simulink model "q_maglev_pid_nominal"  (R2021a)
settings: Solver=ode4  StartTime=0.0  StopTime=inf  FixedStep=5e-4  RelTol=1e-3  AbsTol=1e-6  EnableMultiTasking=on
values from neighbouring files (symbols this model uses):
  IC_MAX = 3    [config_maglev.m]
  K_B = Tb / 4.75    (= 0.00294736842105)    [config_maglev.m]
  Kff_b = ic0 / xb0    [d_maglev_pi_piv.m]
  Ki_c = wn_c^2 * tau_c / Kc_dc    [d_maglev_pi_piv.m]
  Kp_c = (2*zeta_c*wn_c*tau_c - 1) / Kc_dc    [d_maglev_pi_piv.m]
  MAX_XB_WDUP = 1    [setup_maglev.m]
  Rs = 1    [config_maglev.m]
  Tb = 0.014    [config_maglev.m]
  VMAX_AMP = 24    [config_maglev.m]
  xb0 = 6e-3    (= 0.006)    [setup_maglev.m]
  XB_REF_RATE = 5e-3    (= 0.005)    [setup_maglev.m]
undefined symbols (not defined in the file or in its folder): CtunedNom, HIL, qc_get_step_size
libraries: quarc_library x5, pid_lib x1
settings Model: SimulationMode=external  ExtModeTrigDuration=10000  ExtModeAutoUpdateStatusClock=off  Creator=MLevis  LastModifiedBy=MLevis
settings SolverCC: AutoScaleAbsTol=off  AlgebraicLoopSolver=TrustRegion  PositivePriorityOrder=on
settings DataIOCC: SaveFormat=Array  SignalLoggingSaveFormat=ModelDataLogs  ReturnWorkspaceOutputs=off
settings OptimizationCC: BooleanDataType=off  OptimizeBlockIOStorage=off  BufferReuse=off  ExpressionFolding=off  ExpressionDepthLimit=2147483647  LocalBlockOutputs=off  InitFltsAndDblsToZero=on
settings DebuggingCC: SaveWithParameterizedLinksMsg=none  UnderspecifiedInitializationDetection=Classic  MergeDetectMultiDrivingBlocksExec=none  SignalResolutionControl=TryResolveAllWithWarning  MultiTaskDSMMsg=warning  MultiTaskCondExecSysMsg=none  FcnCallInpInsideContextMsg=warning  StateNameClashWarn=warning  SFUnexpectedBacktrackingDiag=warning  SFNoUnconditionalDefaultTransitionDiag=warning  SFExecutionAtInitializationDiag=none  SFMachineParentedDataDiag=warning  ArithmeticOperatorsInVariantConditions=warning
settings HardwareCC: TargetHWDeviceType=32-bit Generic
settings ModelReferenceCC: PropagateSignalLabelsOutOfModel=off
settings SFSimCC: SimUseLocalCustomCode=off  CustomCodeUndefinedFunction=UseInterfaceOnly
settings RTWCC: Description=QUARC Win64 Target Using Toolchain  SystemTargetFile=quarc_win64.tlc  TemplateMakefile=quarc_default_tmf  RTWUseLocalCustomCode=off  Toolchain=QUARC win64 | nmake (64-bit Windows)  BuildConfiguration=Faster Runs
settings CodeAppCC: StateflowObjectComments=on
settings STFCustomTargetCC: ConcurrentExecutionCompliant=on  SystemTargetFile=quarc_win64.tlc
settings GRTTargetCC: TargetLangStandard=C89/C90 (ANSI)  ParMdlRefBuildCompliant=off  CompOptLevelCompliant=off  CombineOutputUpdateFcns=off  MatFileLogging=off  CPPClassGenCompliant=off  GRTInterface=on  ExtMode=on  ExtModeMexFile=quarc_comm
settings ConfigComp: CovMetricSettings=dw  CovSaveCumulativeToWorkspaceVar=on  CovSaveSingleToWorkspaceVar=on  CovExternalEMLEnable=off

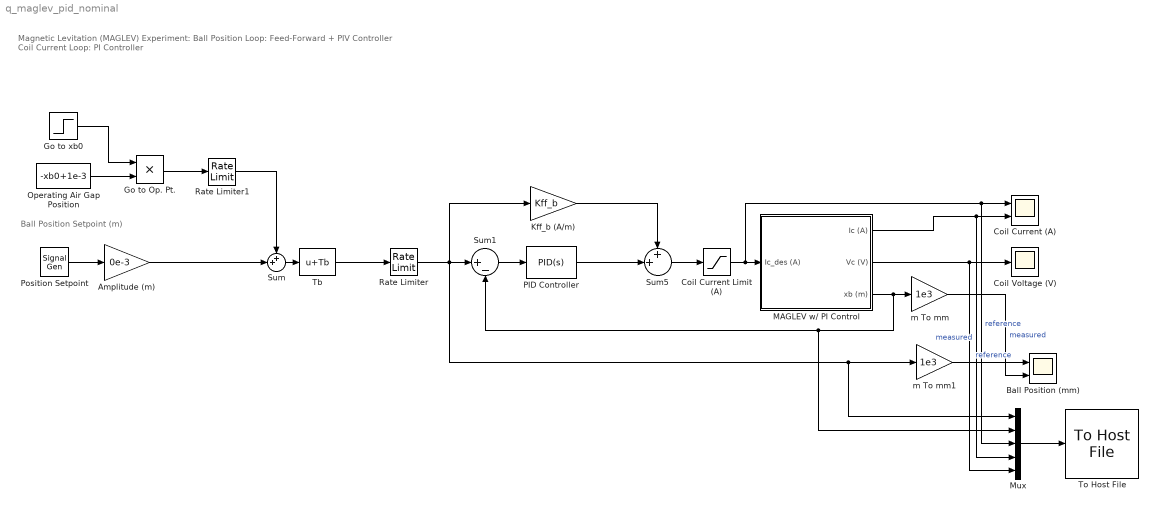
== system q_maglev_pid_nominal ==
  note: Magnetic Levitation (MAGLEV) Experiment:
      | Ball Position Loop: Feed-Forward + PIV Controller
      | Coil Current Loop: PI Controller
  note: Ball Position Setpoint (m)
  Amplitude (m) : Gain  Gain=0e-3  SaturateOnIntegerOverflow=on  OutDataTypeStr=Inherit: Same as input  ParamDataTypeStr=Inherit: Same as input
  Ball Position (mm) : Scope  NumInputPorts=2
  Coil Current Limit (A) : Saturate  UpperLimit=IC_MAX  LowerLimit=0
  Coil Current (A) : Scope  NumInputPorts=2
  Coil Voltage (V) : Scope
  Go to Op. Pt. : Product  RndMeth=Zero
  Go to xb0 : Step  Time=2  SampleTime=0
  Kff_b (A/m) : Gain  Gain=Kff_b  SaturateOnIntegerOverflow=on  OutDataTypeStr=Inherit: Same as input  ParamDataTypeStr=Inherit: Same as input
  MAGLEV w/ PI Control : Subsystem
  Mux : Mux  Inputs=5
  Operating Air Gap Position : Constant  Value=-xb0+1e-3
  PID Controller : pid_lib/PID Controller  Controller=PID  Form=Parallel  TimeDomain=Continuous-time  UseExternalTs=off  SampleTime=-1  IntegratorMethod=Forward Euler  FilterMethod=Forward Euler  ControllerParametersSource=internal  P=CtunedNom.Kp  I=CtunedNom.Ki  D=CtunedNom.Kd  UseFilter=on  N=1/CtunedNom.Tf  TunerSelectOption=Transfer Function Based (PID Tuner App)  InitialConditionSource=internal  InitialConditionForIntegrator=0  InitialConditionForFilter=0  DifferentiatorICPrevScaledInput=0  ExternalReset=none  TrackingMode=off  Kt=1  LimitOutput=on  SatLimitsSource=internal  UpperSaturationLimit=MAX_XB_WDUP  LowerSaturationLimit=-MAX_XB_WDUP  LinearizeAsGain=on  AntiWindupMode=back-calculation  Kb=1  POutMin=[]  POutMax=[]  IOutMin=[]  IOutMax=[]  DOutMin=[]  DOutMax=[]  NOutMin=[]  NOutMax=[]  SumOutMin=[]  SumOutMax=[]  SaturationOutMin=[]  SaturationOutMax=[]  PParamMin=[]  PParamMax=[]  IParamMin=[]  IParamMax=[]  DParamMin=[]  DParamMax=[]  NParamMin=[]  NParamMax=[]  KbParamMin=[]  KbParamMax=[]  KtParamMin=[]  KtParamMax=[]  KbOutMin=[]  KbOutMax=[]  KtOutMin=[]  KtOutMax=[]  IntegratorOutMin=[]  IntegratorOutMax=[]  FilterOutMin=[]  FilterOutMax=[]  SumI1OutMin=[]  SumI1OutMax=[]  SumI2OutMin=[]  SumI2OutMax=[]  SumI3OutMin=[]  SumI3OutMax=[]  SumI4OutMin=[]  SumI4OutMax=[]  SumDOutMin=[]  SumDOutMax=[]  DifferentiatorOutMin=[]  DifferentiatorOutMax=[]  FilterDiffOutCoefMin=[]  FilterDiffOutCoefMax=[]  ReciprocalOutMin=[]  ReciprocalOutMax=[]  SumDenOutMin=[]  SumDenOutMax=[]  SumNumOutMin=[]  SumNumOutMax=[]  DivideOutMin=[]  DivideOutMax=[]  UdiffTsProdOutMin=[]  UdiffTsProdOutMax=[]  NTsProdOutMin=[]  NTsProdOutMax=[]  UintegralTsProdOutMin=[]  UintegralTsProdOutMax=[]  UngainTsProdOutMin=[]  UngainTsProdOutMax=[]  IntegratorContinuousStateAttributes=''  IntegratorStateMustResolveToSignalObject=off  IntegratorRTWStateStorageClass=Auto  FilterContinuousStateAttributes=''  FilterStateMustResolveToSignalObject=off  FilterRTWStateStorageClass=Auto  ParallelPVariant=InternalParameters  IdealPVariant=Disabled  IVariant=InternalParameters  DVariant=InternalParameters  IntegratorVariant=Continuous  SatVariant=Enabled  AWVariant=BackCalculation  PCopyVariant=Disabled  TRVariant=Disabled  FdbkBlocksVariant=Forward  IdealPFdbkVariant=Disabled  SatFdbkVariant=Disabled  DerivativeFilterVariant=ContFilter  NVariant=InternalParameters  NCopyVariant=Disabled  FilterICVariant=InternalICsFilter  IntegratorICVariant=InternalICs  ExternalResetVariant=Disabled  TRSumVariant=Passthrough  SumFdbkVariant=Disabled  SumVariant=Sum_PID  TsampFilterVariant=InternalTs  TsampNgainVariant=Passthrough  TsampIntegralVariant=Passthrough  ExternalSaturationOutDataTypeStr=Inherit: Same as second input
  Position Setpoint : SignalGenerator  WaveForm=square  Frequency=.125
  Rate Limiter : RateLimiter  RisingSlewLimit=XB_REF_RATE  FallingSlewLimit=-XB_REF_RATE
  Rate Limiter1 : RateLimiter  RisingSlewLimit=XB_REF_RATE/4  FallingSlewLimit=-XB_REF_RATE/4  SampleTimeMode=inherited
  Sum : Sum  Inputs=++|
  Sum1 : Sum  Inputs=|+-  InputSameDT=on  SaturateOnIntegerOverflow=on  OutDataTypeStr=Inherit: Same as first input
  Sum5 : Sum  Inputs=++|  InputSameDT=on  SaturateOnIntegerOverflow=on  OutDataTypeStr=Inherit: Same as first input
  Tb : Bias  Bias=Tb
  To Host File : quarc_library/Sinks/To Host/To Host File  file_name=data_maglev_pid_nominal_cntrl.mat  variable_name=data_maglev_cntrl_nom  decimation=1  sample_time=-1  file_format=MAT-file v.4  options=No header or footer  append=off  final_file_name=data_maglev_pid_nominal_cntrl.mat  bitrate=2000000
  m To mm : Gain  Gain=1e3  SaturateOnIntegerOverflow=on  OutDataTypeStr=Inherit: Same as input  ParamDataTypeStr=Inherit: Same as input
  m To mm1 : Gain  Gain=1e3  SaturateOnIntegerOverflow=on  OutDataTypeStr=Inherit: Same as input  ParamDataTypeStr=Inherit: Same as input
  wires:
  Sum1/1 -> PID Controller/1
  MAGLEV w/ PI Control/1(Ic (A)) -> Mux/4, Coil Current (A)/2  "measured"
  Coil Current Limit (A)/1 -> MAGLEV w/ PI Control/1(Ic_des (A)), Mux/3, Coil Current (A)/1  "reference"
  Sum5/1 -> Coil Current Limit (A)/1
  Rate Limiter/1 -> Mux/1, m To mm1/1, Sum1/1, Kff_b (A/m)/1
  Sum/1 -> Tb/1
  MAGLEV w/ PI Control/3(xb (m)) -> Mux/2, Sum1/2, m To mm/1
  Operating Air Gap Position/1 -> Go to Op. Pt./2
  Go to xb0/1 -> Go to Op. Pt./1
  Kff_b (A/m)/1 -> Sum5/1
  Tb/1 -> Rate Limiter/1
  Go to Op. Pt./1 -> Rate Limiter1/1
  m To mm/1 -> Ball Position (mm)/2  "measured"
  MAGLEV w/ PI Control/2(Vc (V)) -> Mux/5, Coil Voltage (V)/1
  m To mm1/1 -> Ball Position (mm)/1  "reference"
  Mux/1 -> To Host File/1
  Position Setpoint/1 -> Amplitude (m)/1
  Amplitude (m)/1 -> Sum/2
  Rate Limiter1/1 -> Sum/1
  PID Controller/1 -> Sum5/2

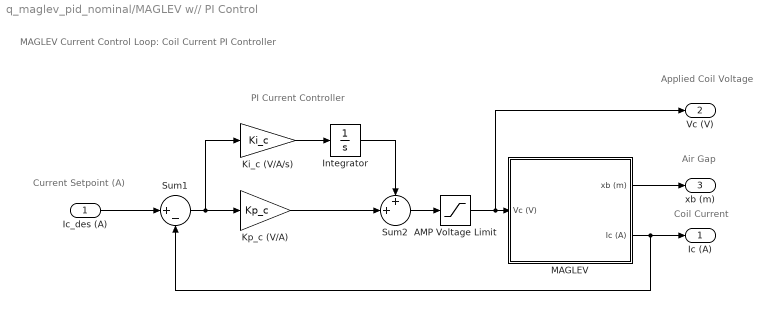
== system q_maglev_pid_nominal/MAGLEV w// PI Control ==
  note: MAGLEV Current Control Loop:
      | Coil Current PI Controller
  note: Current Setpoint (A)
  note: PI Current Controller
  note: Coil Current
  note: Air Gap
  note: Applied Coil Voltage
  Ic_des (A) : Inport
  AMP Voltage Limit : Saturate  UpperLimit=VMAX_AMP  LowerLimit=-VMAX_AMP
  Integrator : Integrator  LimitOutput=on  UpperSaturationLimit=VMAX_AMP  LowerSaturationLimit=-VMAX_AMP
  Ki_c (V/A/s) : Gain  Gain=Ki_c  SaturateOnIntegerOverflow=on  OutDataTypeStr=Inherit: Same as input  ParamDataTypeStr=Inherit: Same as input
  Kp_c (V/A) : Gain  Gain=Kp_c  SaturateOnIntegerOverflow=on  OutDataTypeStr=Inherit: Same as input  ParamDataTypeStr=Inherit: Same as input
  MAGLEV : Subsystem
  Sum1 : Sum  Inputs=|+-  InputSameDT=on  SaturateOnIntegerOverflow=on  OutDataTypeStr=Inherit: Same as first input
  Sum2 : Sum  Inputs=++|  InputSameDT=on  SaturateOnIntegerOverflow=on  OutDataTypeStr=Inherit: Same as first input
  Ic (A) : Outport  InitialOutput=0
  Vc (V) : Outport  Port=2  InitialOutput=0
  xb (m) : Outport  Port=3  InitialOutput=0
  wires:
  Sum1/1 -> Kp_c (V/A)/1, Ki_c (V/A/s)/1
  Kp_c (V/A)/1 -> Sum2/2
  Sum2/1 -> AMP Voltage Limit/1
  Integrator/1 -> Sum2/1
  AMP Voltage Limit/1 -> Vc (V)/1, MAGLEV/1(Vc (V))
  Ic_des (A)/1 -> Sum1/1
  Ki_c (V/A/s)/1 -> Integrator/1
  MAGLEV/1(xb (m)) -> xb (m)/1
  MAGLEV/2(Ic (A)) -> Sum1/2, Ic (A)/1

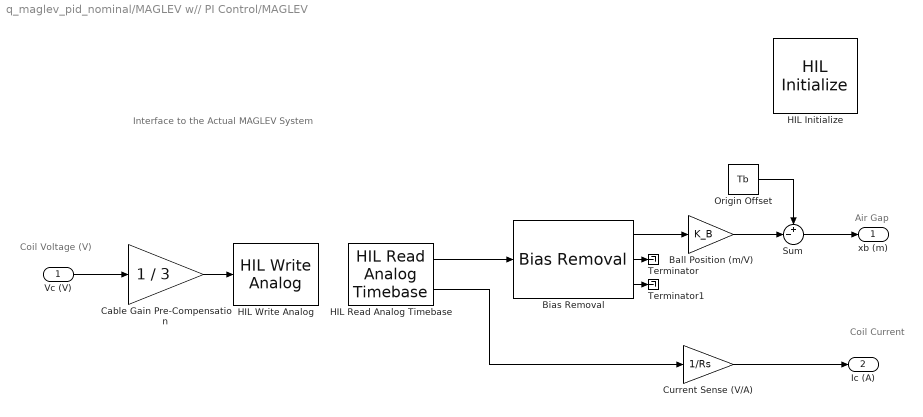
== system q_maglev_pid_nominal/MAGLEV w// PI Control/MAGLEV ==
  note: Interface to the Actual
      | MAGLEV System
  note: Coil Current
  note: Air Gap
  note: Coil Voltage (V)
  Vc (V) : Inport
  Ball Position (m/V) : Gain  Gain=K_B  SaturateOnIntegerOverflow=on  OutDataTypeStr=Inherit: Same as input  ParamDataTypeStr=Inherit: Same as input
  Bias Removal : quarc_library/Discrete/Bias Removal  start_time=0  end_time=0.1  switch_id=0  sample_time=qc_get_step_size
      settings: SourceProductName=QUARC Targets
  Cable Gain Pre-Compensation : Gain  Gain=1 / 3  SaturateOnIntegerOverflow=on  OutDataTypeStr=Inherit: Same as input  ParamDataTypeStr=Inherit: Same as input
  Current Sense (V/A) : Gain  Gain=1/Rs  SaturateOnIntegerOverflow=on  OutDataTypeStr=Inherit: Same as input  ParamDataTypeStr=Inherit: Same as input
  HIL Initialize : quarc_library/Data Acquisition/Generic/Configuration/HIL Initialize  object_name=HIL-1  board_type=q2_usb  board_number=0  board_options=d0=digital;d1=digital;led=auto;update_rate=fast;decimation=1  exclusive=off  active=off  hardware_clocks=[0:2]  clock_modes=[]  initial_clock_frequencies=[]  set_clock_params_at_start=off  set_clock_params_at_switch_in=off  set_clock_frequencies_at_start=off  set_clock_frequencies_at_switch_in=off  analog_input_channels=[0:1]  analog_input_configurations=[]  analog_input_maximums=10  analog_input_minimums=-10  set_analog_input_params_at_start=on  set_analog_input_params_at_switch_in=off  analog_output_channels=[0:1]  analog_output_maximums=10  analog_output_minimums=-10  initial_analog_outputs=[0]  final_analog_outputs=[0]  watchdog_analog_outputs=0  set_analog_output_params_at_start=on  set_analog_output_params_at_switch_in=off  set_analog_outputs_at_start=on  set_analog_outputs_at_switch_in=off  set_analog_outputs_at_terminate=on  set_analog_outputs_at_switch_out=off  set_analog_outputs_on_watchdog=off  digital_input_channels=[]  digital_output_channels=[]  digital_output_configuration=[]  initial_digital_outputs=[1]  final_digital_outputs=[1]  watchdog_digital_outputs=[1]  set_digital_output_params_at_start=off  set_digital_output_params_at_switch_in=off  set_digital_outputs_at_start=on  set_digital_outputs_at_switch_in=off  set_digital_outputs_at_terminate=on  set_digital_outputs_at_switch_out=off  set_digital_outputs_on_watchdog=on  encoder_channels=[0:1]  quadrature=[4]  encoder_filter_frequency=[]  initial_encoder_counts=[0]  set_encoder_params_at_start=on  set_encoder_params_at_switch_in=off  set_encoder_counts_at_start=on  set_encoder_counts_at_switch_in=off  pwm_channels=[]  pwm_modes=[0]  pwm_frequency=1/0.020  pwm_configuration=[]  pwm_alignment=[]  pwm_polarity=[]  pwm_leading_deadband=[]  pwm_trailing_deadband=[]  initial_pwm_outputs=[0]  final_pwm_outputs=[0]  watchdog_pwm_outputs=[0]  set_pwm_params_at_start=on  set_pwm_params_at_switch_in=off  set_pwm_outputs_at_start=on  set_pwm_outputs_at_switch_in=off  set_pwm_outputs_at_terminate=on  set_pwm_outputs_at_switch_out=off  set_pwm_outputs_on_watchdog=off  other_output_channels=[]  initial_other_outputs=[]  final_other_outputs=[]  watchdog_other_outputs=[]  set_other_outputs_at_start=off  set_other_outputs_at_switch_in=off  set_other_outputs_at_terminate=off  set_other_outputs_at_switch_out=off  set_other_outputs_on_watchdog=off
  HIL Read Analog Timebase : quarc_library/Data Acquisition/Generic/Timebases/HIL Read Analog Timebase  object_name=HIL-1  channels=[0:1]  clock=0  active=on  vector_output=off  overflow_mode=Error on overflow  samples_in_buffer=max(ceil(1/qc_get_step_size), 1)
      settings: AttributesFormatString=(%<object_name>)  SourceProductName=QUARC Targets
  HIL Write Analog : quarc_library/Data Acquisition/Generic/Immediate I//O/HIL Write Analog  object_name=HIL-1  channels=0  sample_time=-1  active=off  vector_input=off
  Origin Offset : Constant  Value=Tb
  Sum : Sum  Inputs=+-|
  Terminator : Terminator
  Terminator1 : Terminator
  xb (m) : Outport  InitialOutput=0
  Ic (A) : Outport  Port=2  InitialOutput=0
  wires:
  Current Sense (V/A)/1 -> Ic (A)/1
  Cable Gain Pre-Compensation/1 -> HIL Write Analog/1
  HIL Read Analog Timebase/2 -> Current Sense (V/A)/1
  Origin Offset/1 -> Sum/1
  Ball Position (m/V)/1 -> Sum/2
  Sum/1 -> xb (m)/1
  Vc (V)/1 -> Cable Gain Pre-Compensation/1
  HIL Read Analog Timebase/1 -> Bias Removal/1
  Bias Removal/1 -> Ball Position (m/V)/1
  Bias Removal/2 -> Terminator/1
  Bias Removal/3 -> Terminator1/1
